simulink model "integral_equation"  (R2019b)
settings: Solver=VariableStepAuto  StartTime=0.0  StopTime=10.0  RelTol=1e-3  EnableMultiTasking=on
settings Model: Creator=Administrator  LastModifiedBy=DELL
settings DataIOCC: LimitDataPoints=on  SaveFormat=Array  ReturnWorkspaceOutputs=off
settings OptimizationCC: LifeSpan=inf
settings DebuggingCC: UnderspecifiedInitializationDetection=Classic  MergeDetectMultiDrivingBlocksExec=none  SolverPrmCheckMsg=warning  SFUnexpectedBacktrackingDiag=warning  SFNoUnconditionalDefaultTransitionDiag=warning  SFExecutionAtInitializationDiag=none  ArithmeticOperatorsInVariantConditions=warning
settings HardwareCC: ProdBitPerPointer=32  ProdBitPerSizeT=32  ProdBitPerPtrDiffT=32  ProdLargestAtomicFloat=None  ProdIntDivRoundTo=Undefined  ProdEndianess=Unspecified  ProdWordSize=32  ProdHWDeviceType=32-bit Generic
settings ModelReferenceCC: PropagateSignalLabelsOutOfModel=off
settings SFSimCC: SimUseLocalCustomCode=off  CustomCodeUndefinedFunction=UseInterfaceOnly
settings RTWCC: RTWUseLocalCustomCode=off
settings CodeAppCC: StateflowObjectComments=on
settings GRTTargetCC: TargetLangStandard=C89/C90 (ANSI)
settings ConfigComp: CovMetricSettings=dw  CovHtmlReporting=on  CovSaveCumulativeToWorkspaceVar=on  CovSaveSingleToWorkspaceVar=on  CovExternalEMLEnable=off

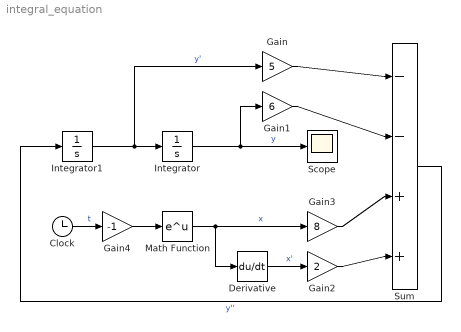
== system integral_equation ==
  Clock : Clock
  Derivative : Derivative
  Gain : Gain  Gain=5
  Gain1 : Gain  Gain=6
  Gain2 : Gain  Gain=2
  Gain3 : Gain  Gain=8
  Gain4 : Gain  Gain=-1
  Integrator : Integrator  InitialCondition=5
      settings: AttributesFormatString=InitVal = %<InitialCondition>
  Integrator1 : Integrator  InitialCondition=-4
      settings: AttributesFormatString=InitVal = %<InitialCondition>
  Math Function : Math  SignedPower=on  SaturateOnIntegerOverflow=on
  Scope : Scope
  Sum : Sum  Inputs=--||++
  wires:
  Integrator1/1 -> Gain/1, Integrator/1  "y'"
  Sum/1 -> Integrator1/1  "y''"
  Integrator/1 -> Gain1/1, Scope/1  "y"
  Clock/1 -> Gain4/1  "t"
  Math Function/1 -> Gain3/1, Derivative/1  "x"
  Derivative/1 -> Gain2/1  "x'"
  Gain2/1 -> Sum/4
  Gain3/1 -> Sum/3
  Gain/1 -> Sum/1
  Gain1/1 -> Sum/2
  Gain4/1 -> Math Function/1
